simulink model "Kalman_Project_save"  (R2023a)
settings: Solver=ode45  StartTime=0  StopTime=25  FixedStep=0.002  RelTol=1e-3  AbsTol=1e-6
values from neighbouring files (symbols this model uses):
  Ts = 0.025    [RL_ABS.m]
undefined symbols (not defined in the file or in its folder): h, J, L, l_f, l_r, m_s, m_t, m_uf, m_ur, Reff, t_brk
libraries: simulink x2, Solver_SF x1, cstblocks x1
settings Model: ExtModeTrigMode=oneshot  Creator=ywata  LastModifiedBy=USER
settings SolverCC: AutoScaleAbsTol=off  AlgebraicLoopSolver=TrustRegion
settings DataIOCC: SaveFormat=Array  SignalLoggingSaveFormat=ModelDataLogs  ReturnWorkspaceOutputs=off  SignalLoggingName=sigsOut
settings OptimizationCC: BlockReduction=off  BooleanDataType=off  ExpressionDepthLimit=2147483647  LifeSpan=inf
settings DebuggingCC: SaveWithParameterizedLinksMsg=none  UnderspecifiedInitializationDetection=Classic  MergeDetectMultiDrivingBlocksExec=none  SignalResolutionControl=TryResolveAllWithWarning  MultiTaskDSMMsg=warning  MultiTaskCondExecSysMsg=none  FcnCallInpInsideContextMsg=warning  UnconnectedInputMsg=warning  UnconnectedOutputMsg=warning  UnconnectedLineMsg=warning  StateNameClashWarn=warning  SFUnexpectedBacktrackingDiag=warning  SFNoUnconditionalDefaultTransitionDiag=warning  SFExecutionAtInitializationDiag=none  ArithmeticOperatorsInVariantConditions=warning
settings HardwareCC: ProdBitPerPointer=32  ProdBitPerSizeT=32  ProdBitPerPtrDiffT=32  ProdLargestAtomicFloat=None  ProdIntDivRoundTo=Undefined  ProdEndianess=Unspecified  ProdWordSize=32  ProdHWDeviceType=32-bit Generic  TargetUnknown=on
settings ModelReferenceCC: PropagateSignalLabelsOutOfModel=off
settings SFSimCC: SimUseLocalCustomCode=off  CustomCodeUndefinedFunction=UseInterfaceOnly
settings RTWCC: TemplateMakefile=grt_vc.tmf  RTWUseLocalCustomCode=off
settings CodeAppCC: StateflowObjectComments=on
settings GRTTargetCC: TargetFcnLib=ansi_tfl_tmw.mat  TargetLangStandard=C89/C90 (ANSI)  CombineOutputUpdateFcns=off  GRTInterface=on
settings ConfigComp: CovMetricSettings=dw  CovSaveCumulativeToWorkspaceVar=on  CovSaveSingleToWorkspaceVar=on  CovExternalEMLEnable=off

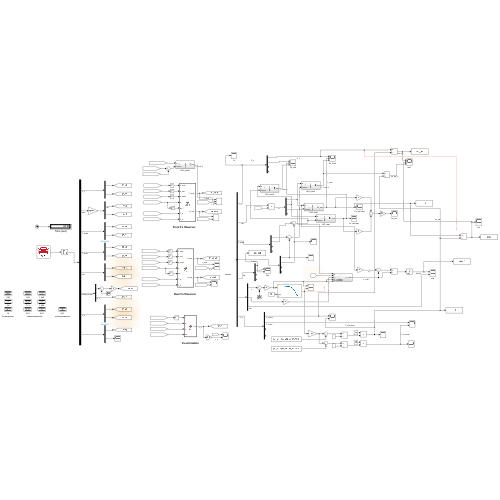
[thumbnail: Simulink's stored preview of the top-level diagram]
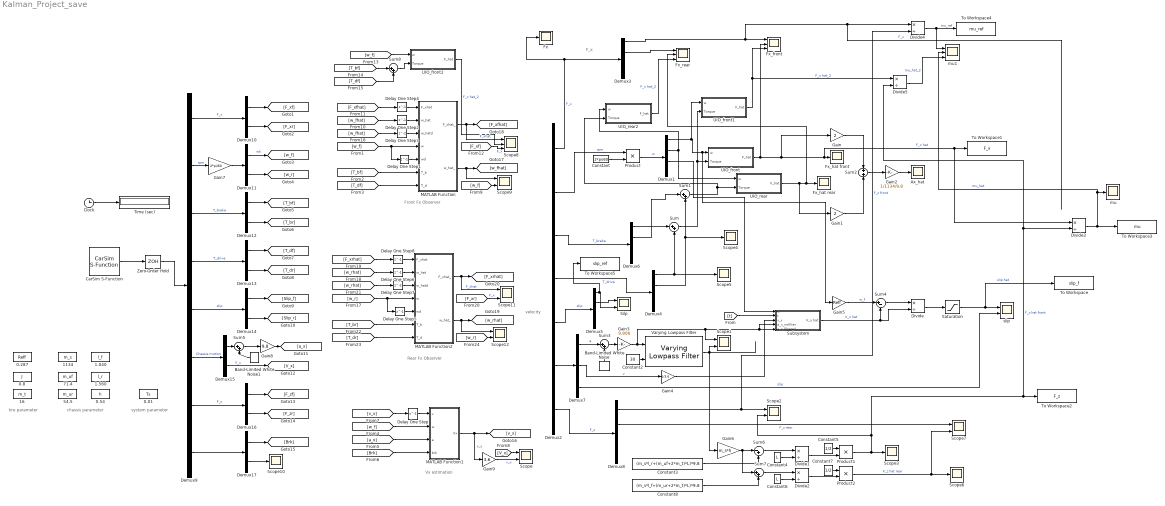
== system Kalman_Project_save ==
  note: Vx estimation
  note: velocity
  note: F_x
  note: chassis parameter
  note: tire parameter
  note: system parameter
  note: Front Fx Observer
  note: Rear Fx Observer
  0.01 : DataStoreMemory  DataStoreName=Ts  WriteAfterWriteMsg=warning  InitialValue=0.01  ShowAdditionalParam=off  OutDataTypeStr=double
  0.287 : DataStoreMemory  DataStoreName=Reff  WriteAfterWriteMsg=warning  InitialValue=0.287  ShowAdditionalParam=off  OutDataTypeStr=double
  0.54 : DataStoreMemory  DataStoreName=h  WriteAfterWriteMsg=warning  InitialValue=0.54  ShowAdditionalParam=off  OutDataTypeStr=double
  0.8 : DataStoreMemory  DataStoreName=J  WriteAfterWriteMsg=warning  InitialValue=0.8  ShowAdditionalParam=off  OutDataTypeStr=double
  1.040 : DataStoreMemory  DataStoreName=l_f  WriteAfterWriteMsg=warning  InitialValue=1.040  ShowAdditionalParam=off  OutDataTypeStr=double
  1.560 : DataStoreMemory  DataStoreName=l_r  WriteAfterWriteMsg=warning  InitialValue=1.560  ShowAdditionalParam=off  OutDataTypeStr=double
  1134 : DataStoreMemory  DataStoreName=m_s  WriteAfterWriteMsg=warning  InitialValue=1134  ShowAdditionalParam=off  OutDataTypeStr=double
  16 : DataStoreMemory  DataStoreName=m_t  WriteAfterWriteMsg=warning  InitialValue=16  ShowAdditionalParam=off  OutDataTypeStr=double
  54.5 : DataStoreMemory  DataStoreName=m_ur  WriteAfterWriteMsg=warning  InitialValue=54.5  ShowAdditionalParam=off  OutDataTypeStr=double
  71.4 : DataStoreMemory  DataStoreName=m_uf  WriteAfterWriteMsg=warning  InitialValue=71.4  ShowAdditionalParam=off  OutDataTypeStr=double
  Ax_hat : Scope
  Band-Limited White Noise : simulink/Sources/Band-Limited White Noise  Cov=[2.25e-8]  Ts=0.01  seed=[23341]
  Band-Limited White Noise1 : simulink/Sources/Band-Limited White Noise  Cov=[2.25e-8]  Ts=0.01  seed=[23341]
  CarSim S-Function : Solver_SF/CarSim S-Function  Priority=1  SIMFILE=simfile.sim  Run_RTs=off  vs_state_ind=Run  StopMode_ind=Vehicle Model
  Clock : Clock
  Constant : Constant  Value=2*pi/60
  Constant2 : Constant  Value=30
  Constant3 : Constant  Value=(m_s*l_r+(m_uf+2*m_t)*L)*9.8
  Constant4 : Constant  Value=L
  Constant5 : Constant  Value=1/2
  Constant6 : Constant  Value=L
  Constant7 : Constant  Value=1/2
  Constant8 : Constant  Value=(m_s*l_f+(m_ur+2*m_t)*L)*9.8
  Delay One Step{,1..2,4..6,8} (7 alike) : Delay  DelayLength=1
  Delay One Step3 : Delay
  Delay One Step7 : Delay
  Demux{1,3..6,8} (6 alike) : Demux  Outputs=[1 1 1 1]
      settings: DisplayOption=none
  Demux{10..17} (8 alike) : Demux  Outputs=[1 1]
      settings: DisplayOption=none
  Demux2 : Demux  Outputs=[4 4 4 4 4 3 4]
      settings: DisplayOption=none
  Demux7 : Demux  Outputs=[1 1 1]
      settings: DisplayOption=none
  Demux9 : Demux  Outputs=[2 2 2 2 2 2 2 2]
      settings: DisplayOption=none
  Divide{,1..5} (6 alike) : Product  Inputs=*/
  Fx : Scope
  Fx_front : Scope  NumInputPorts=3
  Fx_hat front : Scope
  Fx_hat rear : Scope
  Fx_rear : Scope  NumInputPorts=3
  Gain : Gain  Gain=2
  Gain1 : Gain  Gain=2
  Gain2 : Gain  Gain=1/1134/9.8
  Gain3 : Gain  Gain=9.806
  Gain4 : Gain  Gain=1/3.6
  Gain5 : Gain  Gain=Reff
  Gain6 : Gain  Gain=m_s*h
  Gain7 : Gain  Gain=2*pi/60
  Gain8 : Gain  Gain=9.8
  Gain9 : Gain  Gain=3.6
  MATLAB Function : MATLAB Function  TreatAsAtomicUnit=on
  MATLAB Function1 : MATLAB Function  TreatAsAtomicUnit=on
  MATLAB Function2 : MATLAB Function  TreatAsAtomicUnit=on
  Product : Product
  Product1 : Product
  Product2 : Product
  Saturation : Saturate  UpperLimit=1  LowerLimit=-1
  Scope{,1..2,7,9,11..12} (7 alike) : Scope  NumInputPorts=2
  Scope{3..6,10} (5 alike) : Scope
  Scope8 : Scope  NumInputPorts=3
  Silp : Scope  NumInputPorts=2
  Subsystem : Subsystem
  Sum{,1,3,5,7..8} (6 alike) : Sum  Inputs=|++
  Sum2 : Sum  Inputs=+|+
  Sum4 : Sum  Inputs=|+-
  Sum6 : Sum  Inputs=|-+
  Time (sec) : Display
      settings: Format=bank  Decimation=100
  To Workspace : ToWorkspace  VariableName=slip_f  SaveFormat=Timeseries  SampleTime=-1
  To Workspace1 : ToWorkspace  VariableName=F_x  SaveFormat=Timeseries  SampleTime=-1
  To Workspace2 : ToWorkspace  VariableName=F_z  SaveFormat=Timeseries  SampleTime=-1
  To Workspace3 : ToWorkspace  VariableName=mu  SaveFormat=Timeseries  SampleTime=-1
  To Workspace4 : ToWorkspace  VariableName=mu_ref  SaveFormat=Timeseries  SampleTime=-1
  To Workspace5 : ToWorkspace  VariableName=slip_ref  SaveFormat=Timeseries  SampleTime=-1
  UIO_front : Subsystem
  UIO_front1 : Subsystem
  UIO_front2 : Subsystem
  UIO_rear : Subsystem
  UIO_rear2 : Subsystem
  Varying Lowpass Filter : cstblocks/Linear Parameter Varying/Varying Lowpass Filter  N=1
  Zero-Order Hold : ZeroOrderHold  SampleTime=Ts
  mu : Scope
  mu1 : Scope  NumInputPorts=3
  slip : Scope  NumInputPorts=2
  wires:
  Clock/1 -> Time (sec)/1
  Demux2/1 -> Fx/1, Demux3/1  "F_x"
  Demux2/3 -> Demux6/1  "T_brake"
  CarSim S-Function/1 -> Zero-Order Hold/1
  Demux2/2 -> Product/1  "rpm"
  Constant/1 -> Product/2
  Product/1 -> Demux1/1  "w"
  Demux1/2 -> UIO_rear/1(w), UIO_rear2/1(w)
  UIO_rear/1(F_hat) -> Gain1/1, Fx_rear/2, Fx_hat rear/1
  Demux3/1 -> Divide4/1, Fx_front/1  "F_x"
  Demux2/4 -> Demux4/1  "T_drive"
  Demux2/5 -> Demux5/1  "slip"
  Demux3/2 -> Fx_rear/1
  Demux4/2 -> Sum1/2, Scope4/1
  Demux1/1 -> UIO_front1/1(w), Gain5/1, UIO_front/1(w)
  UIO_front/1(F_hat) -> Gain/1, Divide3/1, To Workspace1/1, Fx_hat front/1, Fx_front/2  "F_x hat"
  Demux6/1 -> Sum/1
  Demux4/1 -> Sum/2, Scope5/1
  Sum/1 -> UIO_front1/2(Torque), UIO_front/2(Torque)
  Demux6/2 -> Sum1/1
  Sum1/1 -> UIO_rear2/2(Torque), UIO_rear/2(Torque)
  Gain/1 -> Sum2/1
  Gain1/1 -> Sum2/2
  Sum2/1 -> Gain2/1
  Gain2/1 -> Ax_hat/1
  Demux5/2 -> Silp/1
  Demux5/1 -> To Workspace5/1, Silp/2
  Demux1/3 -> Subsystem/1(w)
  [t] -> Subsystem/2(t)
  Demux2/6 -> Demux7/1
  Varying Lowpass Filter/1 -> Gain6/1, Scope1/2
  Constant2/1 -> Varying Lowpass Filter/2
  Sum3/1 -> Gain3/1
  Demux7/1 -> Sum3/1  "a"
  Demux7/2 -> Gain4/1  "v"
  Gain4/1 -> Subsystem/3(v_x)
  Band-Limited White Noise/1 -> Sum3/2
  Subsystem/1(V_x hat) -> Divide/2, Sum4/2  "V_x hat"
  Gain5/1 -> Sum4/1  "w_f"
  Sum4/1 -> Divide/1
  Divide/1 -> Saturation/1
  Saturation/1 -> To Workspace/1, slip/1  "slip hat"
  Demux7/3 -> slip/2  "slip"
  Demux2/7 -> Demux8/1  "F_z"
  Demux8/2 -> Scope7/1  "F_z rear"
  Demux8/1 -> Divide4/2, Scope2/1  "F_z front"
  Gain6/1 -> Sum7/1, Sum6/1
  Constant3/1 -> Sum6/2
  Sum6/1 -> Divide1/1
  Constant4/1 -> Divide1/2
  Divide1/1 -> Product1/2
  Constant5/1 -> Product1/1
  Product1/1 -> Scope3/1, Divide5/2, Divide3/2, To Workspace2/1, Scope2/2  "F_z hat front"
  Sum7/1 -> Divide2/1
  Constant6/1 -> Divide2/2
  Divide2/1 -> Product2/2
  Constant7/1 -> Product2/1
  Product2/1 -> Scope7/2, Scope6/1  "F_z hat rear"
  Constant8/1 -> Sum7/2
  Gain3/1 -> Scope1/1, Subsystem/4(a_x_nofilter), Subsystem/5(a_x_filtered), Varying Lowpass Filter/1
  Divide3/1 -> mu1/2, mu/1, To Workspace3/1  "mu_hat"
  Divide4/1 -> mu1/1, To Workspace4/1  "mu_ref"
  UIO_front1/1(F_hat) -> Fx_front/3, Divide5/1  "F_x hat_2"
  Divide5/1 -> mu1/3  "mu_hat_2"
  UIO_rear2/1(F_hat) -> Fx_rear/3  "F_x hat_2"
  Zero-Order Hold/1 -> Demux9/1
  Demux9/1 -> Demux10/1  "F_x"
  Demux10/1 -> [F_xf]
  Demux10/2 -> [F_xr]
  Demux11/2 -> [w_r]
  Demux11/1 -> [w_f]  "wk"
  Demux9/2 -> Gain7/1  "rpm"
  Gain7/1 -> Demux11/1
  Demux12/1 -> [T_bf]
  Demux12/2 -> [T_br]
  Demux9/3 -> Demux12/1  "T_brake"
  Demux13/2 -> [T_dr]
  Demux13/1 -> [T_df]
  Demux9/4 -> Demux13/1  "T_drive"
  Demux14/2 -> [Slip_r]
  Demux14/1 -> [Slip_f]
  Demux9/5 -> Demux14/1  "slip"
  Demux15/2 -> [V_x]  "V_x"
  Demux15/1 -> Sum5/1
  Demux9/6 -> Demux15/1  "Chassis motion"
  Demux16/2 -> [F_zr]
  Demux16/1 -> [F_zf]
  Demux9/7 -> Demux16/1  "F_z"
  Band-Limited White Noise1/1 -> Sum5/2
  Sum5/1 -> Gain8/1
  Gain8/1 -> [a_x]
  [w_f] -> MATLAB Function1/2(w)
  [a_x] -> MATLAB Function1/3(a)
  [Brk] -> MATLAB Function1/4(brk)
  Demux9/8 -> Demux17/1
  MATLAB Function1/1(Vx) -> Gain9/1, [v_x]  "v_x"
  [v_x] -> Delay One Step/1
  Delay One Step/1 -> MATLAB Function1/1(v)
  Gain9/1 -> Scope/2  "v_x"
  [V_x] -> Scope/1
  Delay One Step1/1 -> MATLAB Function/5(wd)
  [w_f] -> MATLAB Function/4(w), Delay One Step1/1
  MATLAB Function/2(w_hat_) -> Scope9/1, [w_fhat]
  Delay One Step3/1 -> MATLAB Function/3(w_hatd)
  MATLAB Function/1(F_xhat_) -> Scope8/1, [F_xfhat]  "F_xhat"
  [F_xfhat] -> Delay One Step4/1
  [F_xf] -> Scope8/3  "F_x"
  [w_fhat] -> Delay One Step2/1
  Delay One Step2/1 -> MATLAB Function/2(w_hat)
  Delay One Step4/1 -> MATLAB Function/1(F_xhat)
  Demux17/1 -> [Brk]
  Demux17/2 -> Scope10/1
  [w_f] -> Scope9/2
  [T_bf] -> MATLAB Function/6(T_b)
  [T_df] -> MATLAB Function/7(T_d)
  [w_f] -> UIO_front2/1(w)
  [T_bf] -> Sum8/1
  [T_df] -> Sum8/2
  Sum8/1 -> UIO_front2/2(Torque)
  UIO_front2/1(F_hat) -> Scope8/2  "F_x hat_2"
  [w_fhat] -> Delay One Step3/1
  Delay One Step8/1 -> MATLAB Function2/1(F_xhat)
  MATLAB Function2/1(F_xhat_) -> Scope11/1, [F_xrhat]  "F_xhat"
  [F_xr] -> Scope11/2  "F_x"
  [w_rhat] -> Delay One Step6/1
  Delay One Step7/1 -> MATLAB Function2/3(w_hatd)
  [w_rhat] -> Delay One Step7/1
  [F_xrhat] -> Delay One Step8/1
  [w_r] -> Scope12/2
  [T_dr] -> MATLAB Function2/7(T_d)
  [w_r] -> MATLAB Function2/4(w), Delay One Step5/1
  MATLAB Function2/2(w_hat_) -> Scope12/1, [w_rhat]
  Delay One Step6/1 -> MATLAB Function2/2(w_hat)
  [T_br] -> MATLAB Function2/6(T_b)
  Delay One Step5/1 -> MATLAB Function2/5(wd)

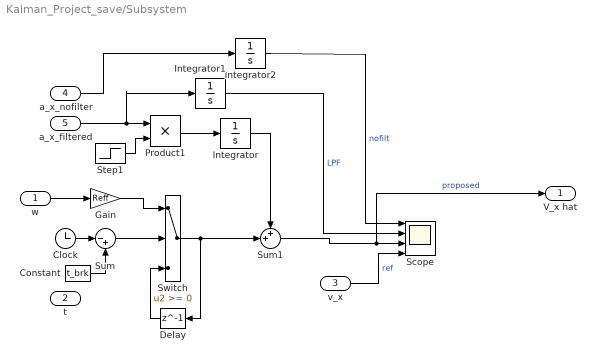
== system Kalman_Project_save/Subsystem ==
  w : Inport
  t : Inport  Port=2
  v_x : Inport  Port=3
  a_x_nofilter : Inport  Port=4
  a_x_filtered : Inport  Port=5
  Clock : Clock
  Constant : Constant  Value=t_brk
  Delay : Delay  DelayLength=1  InitialCondition=0
  Gain : Gain  Gain=Reff
  Integrator : Integrator
  Integrator1 : Integrator
  Integrator2 : Integrator
  Product1 : Product
  Scope : Scope  NumInputPorts=4
  Step1 : Step  Time=t_brk  SampleTime=0
  Sum : Sum  Inputs=|-+
  Sum1 : Sum  Inputs=++|
  Switch : Switch  SaturateOnIntegerOverflow=off  InputSameDT=off
  V_x hat : Outport
  wires:
  w/1 -> Gain/1
  Gain/1 -> Switch/1
  a_x_filtered/1 -> Integrator1/1, Product1/1
  v_x/1 -> Scope/4  "ref"
  Step1/1 -> Product1/2
  Product1/1 -> Integrator/1
  Integrator1/1 -> Scope/2  "LPF"
  Clock/1 -> Sum/1
  Switch/1 -> Sum1/2, Delay/1
  Delay/1 -> Switch/3
  Constant/1 -> Sum/2
  Sum/1 -> Switch/2
  Integrator/1 -> Sum1/1
  Sum1/1 -> V_x hat/1, Scope/3  "proposed"
  a_x_nofilter/1 -> Integrator2/1
  Integrator2/1 -> Scope/1  "nofilt"

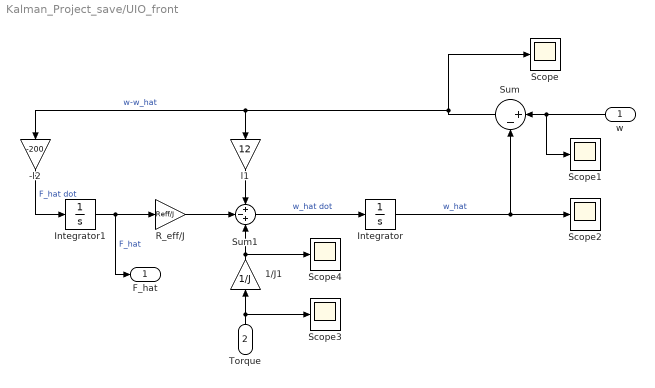
== system Kalman_Project_save/UIO_front ==
  w : Inport
  Torque : Inport  Port=2
  -l2 : Gain  Gain=-200
  1/J1 : Gain  Gain=1/J
  Integrator : Integrator
  Integrator1 : Integrator
  R_eff/J : Gain  Gain=Reff/J
  Scope{,1..4} (5 alike) : Scope
  Sum : Sum  Inputs=|+-
  Sum1 : Sum  Inputs=+-+
  l1 : Gain  Gain=12
  F_hat : Outport
  wires:
  w/1 -> Scope1/1, Sum/1
  Integrator/1 -> Sum/2, Scope2/1  "w_hat"
  Sum1/1 -> Integrator/1  "w_hat dot"
  Sum/1 -> l1/1, -l2/1, Scope/1  "w-w_hat"
  l1/1 -> Sum1/1
  -l2/1 -> Integrator1/1  "F_hat dot"
  Integrator1/1 -> F_hat/1, R_eff/J/1  "F_hat"
  R_eff/J/1 -> Sum1/2
  Torque/1 -> 1/J1/1, Scope3/1
  1/J1/1 -> Sum1/3, Scope4/1

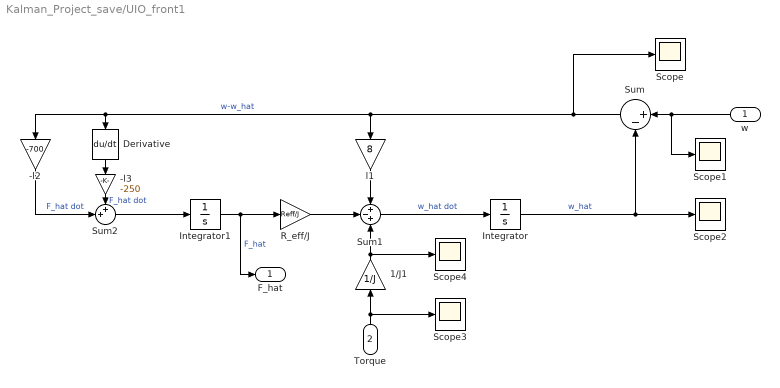
== system Kalman_Project_save/UIO_front1 ==
  w : Inport
  Torque : Inport  Port=2
  -l2 : Gain  Gain=-700
  -l3 : Gain  Gain=-250
  1/J1 : Gain  Gain=1/J
  Derivative : Derivative
  Integrator : Integrator
  Integrator1 : Integrator
  R_eff/J : Gain  Gain=Reff/J
  Scope{,1..4} (5 alike) : Scope
  Sum : Sum  Inputs=|+-
  Sum1 : Sum  Inputs=+-+
  Sum2 : Sum  Inputs=++|
  l1 : Gain  Gain=8
  F_hat : Outport
  wires:
  w/1 -> Scope1/1, Sum/1
  Integrator/1 -> Sum/2, Scope2/1  "w_hat"
  Sum1/1 -> Integrator/1  "w_hat dot"
  Sum/1 -> -l2/1, Derivative/1, l1/1, Scope/1  "w-w_hat"
  l1/1 -> Sum1/1
  -l2/1 -> Sum2/2  "F_hat dot"
  Integrator1/1 -> F_hat/1, R_eff/J/1  "F_hat"
  R_eff/J/1 -> Sum1/2
  Torque/1 -> 1/J1/1, Scope3/1
  1/J1/1 -> Sum1/3, Scope4/1
  Sum2/1 -> Integrator1/1
  Derivative/1 -> -l3/1
  -l3/1 -> Sum2/1  "F_hat dot"

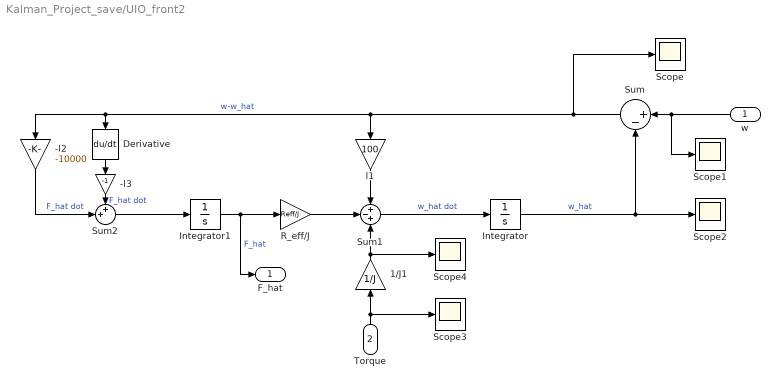
== system Kalman_Project_save/UIO_front2 ==
  w : Inport
  Torque : Inport  Port=2
  -l2 : Gain  Gain=-10000
  -l3 : Gain  Gain=-1
  1/J1 : Gain  Gain=1/J
  Derivative : Derivative
  Integrator : Integrator
  Integrator1 : Integrator
  R_eff/J : Gain  Gain=Reff/J
  Scope{,1..4} (5 alike) : Scope
  Sum : Sum  Inputs=|+-
  Sum1 : Sum  Inputs=+-+
  Sum2 : Sum  Inputs=++|
  l1 : Gain  Gain=100
  F_hat : Outport
  wires:
  w/1 -> Scope1/1, Sum/1
  Integrator/1 -> Sum/2, Scope2/1  "w_hat"
  Sum1/1 -> Integrator/1  "w_hat dot"
  Sum/1 -> -l2/1, Derivative/1, l1/1, Scope/1  "w-w_hat"
  l1/1 -> Sum1/1
  -l2/1 -> Sum2/2  "F_hat dot"
  Integrator1/1 -> F_hat/1, R_eff/J/1  "F_hat"
  R_eff/J/1 -> Sum1/2
  Torque/1 -> 1/J1/1, Scope3/1
  1/J1/1 -> Sum1/3, Scope4/1
  Sum2/1 -> Integrator1/1
  Derivative/1 -> -l3/1
  -l3/1 -> Sum2/1  "F_hat dot"

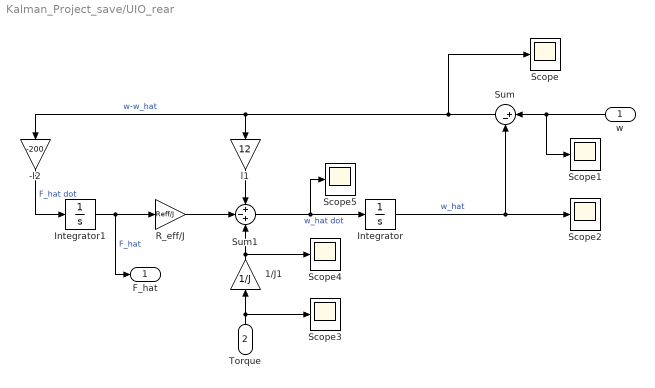
== system Kalman_Project_save/UIO_rear ==
  w : Inport
  Torque : Inport  Port=2
  -l2 : Gain  Gain=-200
  1/J1 : Gain  Gain=1/J
  Integrator : Integrator
  Integrator1 : Integrator
  R_eff/J : Gain  Gain=Reff/J
  Scope{,1..5} (6 alike) : Scope
  Sum : Sum  Inputs=|+-
  Sum1 : Sum  Inputs=+-+
  l1 : Gain  Gain=12
  F_hat : Outport
  wires:
  w/1 -> Scope1/1, Sum/1
  Integrator/1 -> Sum/2, Scope2/1  "w_hat"
  Sum1/1 -> Scope5/1, Integrator/1  "w_hat dot"
  Sum/1 -> Scope/1, -l2/1, l1/1  "w-w_hat"
  l1/1 -> Sum1/1
  -l2/1 -> Integrator1/1  "F_hat dot"
  Integrator1/1 -> F_hat/1, R_eff/J/1  "F_hat"
  R_eff/J/1 -> Sum1/2
  Torque/1 -> 1/J1/1, Scope3/1
  1/J1/1 -> Sum1/3, Scope4/1

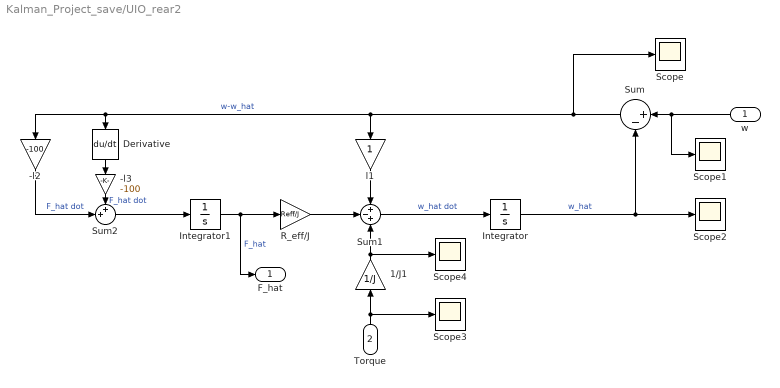
== system Kalman_Project_save/UIO_rear2 ==
  w : Inport
  Torque : Inport  Port=2
  -l2 : Gain  Gain=-100
  -l3 : Gain  Gain=-100
  1/J1 : Gain  Gain=1/J
  Derivative : Derivative
  Integrator : Integrator
  Integrator1 : Integrator
  R_eff/J : Gain  Gain=Reff/J
  Scope{,1..4} (5 alike) : Scope
  Sum : Sum  Inputs=|+-
  Sum1 : Sum  Inputs=+-+
  Sum2 : Sum  Inputs=++|
  l1 : Gain
  F_hat : Outport
  wires:
  w/1 -> Scope1/1, Sum/1
  Integrator/1 -> Sum/2, Scope2/1  "w_hat"
  Sum1/1 -> Integrator/1  "w_hat dot"
  Sum/1 -> -l2/1, Derivative/1, l1/1, Scope/1  "w-w_hat"
  l1/1 -> Sum1/1
  -l2/1 -> Sum2/2  "F_hat dot"
  Integrator1/1 -> F_hat/1, R_eff/J/1  "F_hat"
  R_eff/J/1 -> Sum1/2
  Torque/1 -> 1/J1/1, Scope3/1
  1/J1/1 -> Sum1/3, Scope4/1
  Sum2/1 -> Integrator1/1
  Derivative/1 -> -l3/1
  -l3/1 -> Sum2/1  "F_hat dot"

== matlab function Kalman_Project_save/MATLAB Function1 ==
  data: v input; w input; Vx output; a input; brk input; Reff data_store_memory; Ts data_store_memory
function Vx = fcn(v,w,a,brk)
global Ts Reff;

if brk == 0
    Vx = (w*Reff + v)/2;
else
    Vx = v + a*Ts;
end
end

== matlab function Kalman_Project_save/MATLAB Function ==
  data: F_xhat input; F_xhat_ output; w_hat input; w_hatd input; w_hat_ output; w input; wd input; T_b input; T_d input; Reff data_store_memory; J data_store_memory; Ts data_store_memory
function [F_xhat_,w_hat_]= UIO_f(F_xhat,w_hat,w_hatd,w,wd,T_b,T_d)

global Reff J Ts;
l1 = 1; l2 = 1000; l3 = 200;

w_hatdot = 1/J*(T_b+T_d) - Reff/J*F_xhat + l1*(w-w_hat);
w_hat_ = w_hat + w_hatdot*Ts;

F_xhatdot = -l2*(w-w_hat) - l3*((w-wd)/Ts - (w_hat-w_hatd)/Ts);
F_xhat_ = F_xhat + F_xhatdot*Ts;




end

== matlab function Kalman_Project_save/MATLAB Function2 ==
  data: F_xhat input; F_xhat_ output; w_hat input; w_hatd input; w_hat_ output; w input; wd input; T_b input; T_d input; Reff data_store_memory; J data_store_memory; Ts data_store_memory
function [F_xhat_,w_hat_]= UIO_f(F_xhat,w_hat,w_hatd,w,wd,T_b,T_d)

global Reff J Ts;
l1 = 1; l2 = 1000; l3 = 200;

w_hatdot = 1/J*(T_b+T_d) - Reff/J*F_xhat + l1*(w-w_hat);
w_hat_ = w_hat + w_hatdot*Ts;

F_xhatdot = -l2*(w-w_hat) - l3*((w-wd)/Ts - (w_hat-w_hatd)/Ts);
F_xhat_ = F_xhat + F_xhatdot*Ts;




end
